simulink model "model_base_bros_r2016b"  (R2016b)
settings: Solver=FixedStepDiscrete  StartTime=0.0  StopTime=inf  FixedStep=sampleTime  RelTol=1e-3
PostLoadFcn:
  | % load model parameters
  | % pname = fileparts(get_param('model_base_bros','filename'));
  | % run([pname  '\parameters_base_model_bros.m']);
  | parameters_base_model_bros;
  | 
  | % set requested state
  | set_param('model_base_bros_r2016b/Requested state','Value',num2str(0));
InitFcn:
  | % load model parameters
  | % pname = fileparts(get_param('model_base_bros','filename'));
  | % run([pname  '\parameters_base_model_bros.m']);
  | parameters_base_model_bros;
  | 
  | % set requested state
  | set_param('model_base_bros_r2016b/Requested state','Value',num2str(0));
StartFcn:
  | % load model parameters
  | % pname = fileparts(get_param('model_base_bros','filename'));
  | % run([pname  '\parameters_base_model_bros.m']);
  | parameters_base_model_bros;
  | 
  | % set requested state
  | set_param('model_base_bros_r2016b/Requested state','Value',num2str(0));
StopFcn:
  | % switch off data logger (to hopefully avoid corrupt files). TwinCAT doesn't properly switch off the logger when shutting down the model
  | % no idea if this'll work.
  | set_param('model_base_bros_r2016b/Record data (1 = yes, 0 = no)','Value',num2str(0));
values from neighbouring files (symbols this model uses):
  FFMatrix = -[0 -15; 15 0]    [parameters_base_model_bros.m]
  Lb = 0.07    [parameters_base_model_bros.m]
  Lf = 0.238    [parameters_base_model_bros.m]
  Lu = 0.153    [parameters_base_model_bros.m]
  msin_data_dist1 = [5 11 19 41 59 71 101 137 179 227 0.0358569687947 0.0275584886584 ... (30 elements, 10x3)]    [forcingfunction_data_id.mat]    (also in forcingfunction_data_id_2d_var6_1.mat = [0 0 0 0 0 0 0 0 0 0 0 0 ... (60 elements, 10x6)]; forcingfunction_data_id_2d_var75_nt11.mat = [0 0 0 0 0 0 0 0 0 0 0 0 ... (60 elements, 10x6)]; forcingfunction_data_id_nt10_var6.mat = [5 11 19 41 59 71 101 137 179 227 0.0248424367031 0.01909308)
  msin_data_dist2 = [7 13 23 43 61 73 103 139 181 229 0.0366642780879 0.0272817537998 ... (30 elements, 10x3)]    [forcingfunction_data_id.mat]    (also in forcingfunction_data_id_2d_var6_1.mat = [0 0 0 0 0 0 0 0 0 0 0 0 ... (60 elements, 10x6)]; forcingfunction_data_id_2d_var75_nt11.mat = [0 0 0 0 0 0 0 0 0 0 0 0 ... (60 elements, 10x6)]; forcingfunction_data_id_nt10_var6.mat = [7 13 23 43 61 73 103 139 181 229 0.0254017569884 0.01890135)
  msin_data_target = [2 9 17 27 37 47 0.0347382902327 0.0275101923829 0.0180185190239 0.0110214159229 0.0075682474126 0.00574660779142 ... (18 elements, 6x3)]    [forcingfunction_data_id.mat]    (also in forcingfunction_data_id_2d_var6_1.mat = [5 11 23 37 51 71 101 137 171 226 0.0252651788023 0.01941798; forcingfunction_data_id_2d_var75_nt11.mat = [5 11 23 37 51 71 101 137 173 227 263 0.0282088788597 ... (6; forcingfunction_data_id_nt10_var6.mat = [2 9 17 29 37 47 67 107 149 211 0.0239780224904 0.0189888450; forcingfunction_id_emg.mat = [3 7 13 19 31 0.0450441024419 0.0275859409824 0.015205627144)
  sampleTime = 0.001    [parameters_base_model_bros.m]
  Tm = 81.92    [forcingfunction_data_id_2d_var6_1.mat]    (also in forcingfunction_data_id_2d_var75_nt11.mat; forcingfunction_data_id_nt10_var6.mat; forcingfunction_id_emg.mat = 24)
undefined symbols (not defined in the file or in its folder): BROS1, BROS2
libraries: simulink x28, LibraryFM x14, VariousBlocksLibrary x13, simulink_extras x1
(part 4 of 4)

== matlab function model_base_bros_r2016b/Experiment & Haptics/ msin_disturbance2 ==
  data: time input; T input; time_rand input; msin_data input; p output; v output; a output; Tm input
function [p, v, a]  = msin (time, T, time_rand, msin_data,Tm) 

n = msin_data(:,1);
A = msin_data(:,2);
ph = msin_data(:,3);

% prepare frequencies
dw = 2*pi/Tm; %w0 depends on trial duration
w = dw*n;

% calculate position, velocity, acceleration
p = 0;
v = 0;
a = 0;

% randomization
% for every multiple of 20, rotate the target signal
% nRand = floor(time_rand/T);
% if nRand > 5, nRand = 5; end

% % add random starting time (semi-randomization)
time = time + mod(time_rand,T);

% calculate sum-of-sines
for i = 1:length(w)
    % position
    p = p + A(i)*sin(w(i)*time+ph(i));
    
    % velocity
    v = v + A(i)*w(i)*cos(w(i)*time+ph(i));
     
    % velocity
    a = a - A(i)*w(i)^2*sin(w(i)*time+ph(i));
end

% due to the difference in coordiante systems (of human reaching, y
% forward, x to the right; robot: y towards you and x to the left), rotate
% the target such that it is in a human-centered coordinate system.
p = -p;
v = -v;
a = -a;

% % rotate target (to make it more random-appearing)
% thetaRot = nRand*(2*pi/6);
% 
% R = [cos(thetaRot) -sin(thetaRot); sin(thetaRot) cos(thetaRot)];
% 
% p = R*p;
% v = R*v;
% a = R*a;

end
